simulink model "Ques1"  (R2020b)
settings: Solver=VariableStepAuto  StartTime=0.0  StopTime=100  RelTol=1e-3
undefined symbols (not defined in the file): b, K1, K12, M1, M2
settings Model: Creator=hp  LastModifiedBy=hp

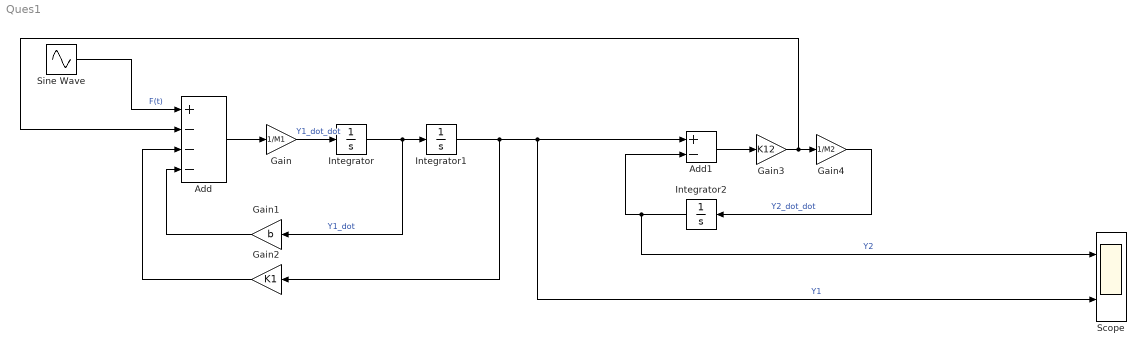
== system Ques1 ==
  Add : Sum  Inputs=+---
  Add1 : Sum  Inputs=+-
  Gain : Gain  Gain=1/M1
  Gain1 : Gain  Gain=b
  Gain2 : Gain  Gain=K1
  Gain3 : Gain  Gain=K12
  Gain4 : Gain  Gain=1/M2
  Integrator : Integrator
  Integrator1 : Integrator
  Integrator2 : Integrator
  Scope : Scope  NumInputPorts=2
  Sine Wave : Sin  Amplitude=2  Frequency=2*pi*10  SampleTime=0
  wires:
  Integrator/1 -> Gain1/1, Integrator1/1  "Y1_dot"
  Add/1 -> Gain/1
  Integrator1/1 -> Scope/2, Add1/1, Gain2/1  "Y1"
  Sine Wave/1 -> Add/1  "F(t)"
  Gain/1 -> Integrator/1  "Y1_dot_dot"
  Gain1/1 -> Add/4
  Gain2/1 -> Add/3
  Integrator2/1 -> Scope/1, Add1/2  "Y2"
  Add1/1 -> Gain3/1
  Gain3/1 -> Add/2, Gain4/1
  Gain4/1 -> Integrator2/1  "Y2_dot_dot"
